simulink model "Week1_Q4"  (R2020b)
settings: Solver=VariableStepAuto  StartTime=0.0  StopTime=10.0  RelTol=1e-3
settings Model: Creator=vikas  LastModifiedBy=vikas

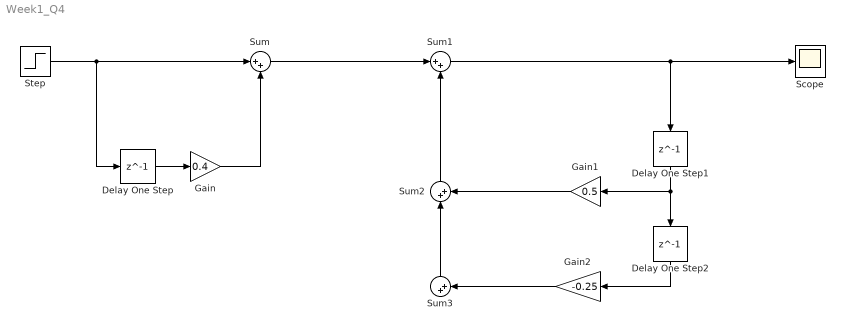
== system Week1_Q4 ==
  Delay One Step : Delay  DelayLength=1
  Delay One Step1 : Delay  DelayLength=1
  Delay One Step2 : Delay  DelayLength=1
  Gain : Gain  Gain=0.4
  Gain1 : Gain  Gain=0.5
  Gain2 : Gain  Gain=-0.25
  Scope : Scope
  Step : Step  SampleTime=0
  Sum{,1..3} (4 alike) : Sum  Inputs=|++
  wires:
  Sum/1 -> Sum1/1
  Delay One Step2/1 -> Gain2/1
  Step/1 -> Sum/1, Delay One Step/1
  Gain1/1 -> Sum2/2
  Sum1/1 -> Delay One Step1/1, Scope/1
  Gain/1 -> Sum/2
  Delay One Step/1 -> Gain/1
  Delay One Step1/1 -> Delay One Step2/1, Gain1/1
  Gain2/1 -> Sum3/2
  Sum3/1 -> Sum2/1
  Sum2/1 -> Sum1/2
